simulink model "xpccanpcififo2"  (Simulink 4.00)
settings: Solver=FixedStepDiscrete  StartTime=0.0  StopTime=inf  RelTol=1e-3
libraries: xpclib x14, simulink3 x1
settings Model: Creator=mvetsch  LastModifiedBy=mvetsch  SimulationMode=external  RTWSystemTargetFile=xpctarget.tlc  RTWOptions="-aExtMode=1 -aForceParamTrailComments=0 -aInlineInvariantSignals=0 -aInlineParameters=0 -aLocalBlockOutputs=0 -aRL32IRQSourceModifier=\"Timer\" -aRL32LogBufSizeModifier=100000 -aRL32LogTETModifier=1 -aRL32ModeModifier=\"Real-Time\" -aRL32ObjectName=\"tg\" -aRL32ScopeModifier=1 -aRTWVerbose=1 -aRollThreshold=5 -aShowEliminatedStatements=1"  RTWTemplateMakefile=xpc_default_tmf  ExtModeMexFile=ext_xpc  ExtModeArmWhenConnect=off  OptimizeBlockIOStorage=off  BlockReductionOpt=off

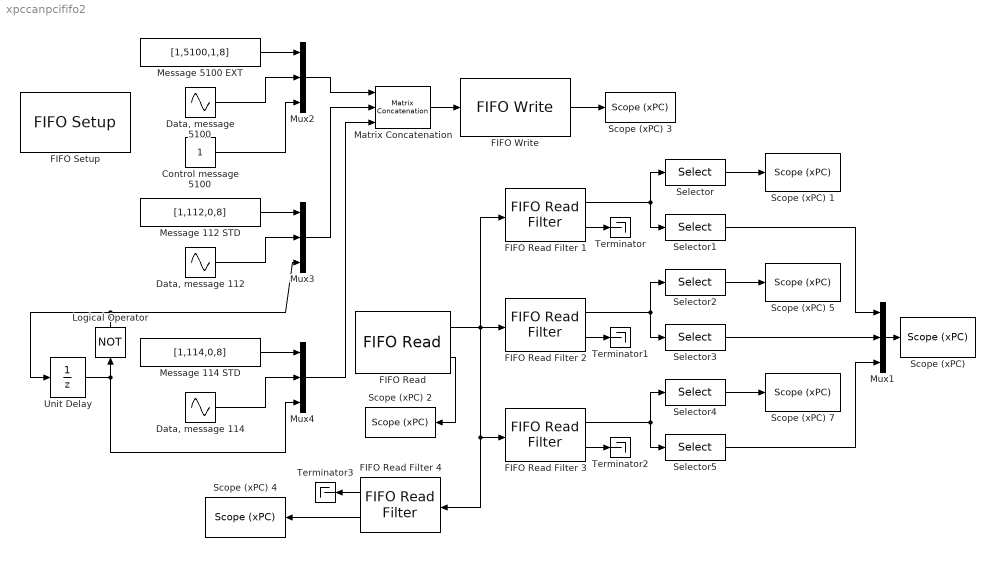
== system xpccanpcififo2 ==
  Control message 5100 : Constant  Value=1  VectorParams1D=off
  "Data, message 112" : Sin  Amplitude=2  Frequency=20*2*pi  Phase=0  SampleTime=0.001
  "Data, message 114" : Sin  Amplitude=3  Frequency=20*2*pi  Phase=0  SampleTime=0.001
  "Data, message 5100" : Sin  Amplitude=1  Frequency=20*2*pi  Phase=0  SampleTime=0.001
  "FIFO Read " : xpclib/CAN/Softing/CAN-AC2-PCI SJA 1000/FIFO Mode/FIFO Read   board=1  depth=3  status=on  sampletime=0.001
  FIFO Read Filter 1 : xpclib/CAN/Softing/CAN-AC2-PCI SJA 1000/FIFO Mode/FIFO Read Filter   portin=2  ctypein=EDF  direction=Include  ident=[5100]  identsel=Include
  FIFO Read Filter 2 : xpclib/CAN/Softing/CAN-AC2-PCI SJA 1000/FIFO Mode/FIFO Read Filter   portin=2  ctypein=SDF  direction=Include  ident=[112]  identsel=Include
  FIFO Read Filter 3 : xpclib/CAN/Softing/CAN-AC2-PCI SJA 1000/FIFO Mode/FIFO Read Filter   portin=2  ctypein=SDF  direction=Include  ident=[114]  identsel=Include
  FIFO Read Filter 4 : xpclib/CAN/Softing/CAN-AC2-PCI SJA 1000/FIFO Mode/FIFO Read Filter   Orientation=left  portin=2  ctypein=NE  direction=Include  ident=[]  identsel=Include
  "FIFO Setup " : xpclib/CAN/Softing/CAN-AC2-PCI SJA 1000/FIFO Mode/FIFO Setup   board=1  can1bus=Highspeed (ISO 11898)  can1Baudrate=1 MBaud  can1UserBR=[1,1,4,3]  acc1=[0,0,0,0]  can2bus=Highspeed (ISO 11898)  can2Baudrate=1 MBaud  can2UserBR=[1,1,4,3]  acc2=[0,0,0,0]  efdetection=off  init=[]  term=[]  ioBaseAddress=-1
  "FIFO Write " : xpclib/CAN/Softing/CAN-AC2-PCI SJA 1000/FIFO Mode/FIFO Write   board=1  status=on  sampletime=-1
  Logical Operator : Logic  Orientation=up  Operator=NOT  Inputs=2
  Matrix Concatenation : simulink3/Signals & Systems/Matrix Concatenation  numInports=3  catMethod=Vertical
  Message 112 STD : Constant  Value=[1,112,0,8]  VectorParams1D=off
  Message 114 STD : Constant  Value=[1,114,0,8]  VectorParams1D=off
  Message 5100 EXT : Constant  Value=[1,5100,1,8]  VectorParams1D=off
  Mux{1..4} (4 alike) : Mux  Inputs=3
  "Scope (xPC) " : xpclib/Misc./Scope (xPC)   scopeno=3  scopetype=Target  viewmode=Graphical redraw  grid=on  ylimits=[0,0]  autostart=on  nosamples=100  noprepostsamples=0  interleave=1  triggermode=FreeRun  triggersignal=1  triggerlevel=0.0  triggerslope=either  triggerscope=1
  Scope (xPC) 1 : xpclib/Misc./Scope (xPC)   scopeno=4  scopetype=Target  viewmode=Numerical  grid=on  ylimits=[0,0]  autostart=on  nosamples=3  noprepostsamples=0  interleave=1  triggermode=FreeRun  triggersignal=1  triggerlevel=0.0  triggerslope=either  triggerscope=1
  Scope (xPC) 2 : xpclib/Misc./Scope (xPC)   Orientation=left  scopeno=2  scopetype=Target  viewmode=Numerical  grid=on  ylimits=[0,0]  autostart=on  nosamples=3  noprepostsamples=0  interleave=1  triggermode=FreeRun  triggersignal=1  triggerlevel=0.0  triggerslope=either  triggerscope=1
  Scope (xPC) 3 : xpclib/Misc./Scope (xPC)   scopeno=1  scopetype=Target  viewmode=Numerical  grid=on  ylimits=[0,0]  autostart=on  nosamples=3  noprepostsamples=0  interleave=1  triggermode=FreeRun  triggersignal=1  triggerlevel=0.0  triggerslope=either  triggerscope=1
  Scope (xPC) 4 : xpclib/Misc./Scope (xPC)   Orientation=left  scopeno=7  scopetype=Target  viewmode=Numerical  grid=on  ylimits=[0,0]  autostart=on  nosamples=3  noprepostsamples=0  interleave=1  triggermode=FreeRun  triggersignal=1  triggerlevel=0.0  triggerslope=either  triggerscope=1
  Scope (xPC) 5 : xpclib/Misc./Scope (xPC)   scopeno=5  scopetype=Target  viewmode=Numerical  grid=on  ylimits=[0,0]  autostart=on  nosamples=3  noprepostsamples=0  interleave=1  triggermode=FreeRun  triggersignal=1  triggerlevel=0.0  triggerslope=either  triggerscope=1
  Scope (xPC) 7 : xpclib/Misc./Scope (xPC)   scopeno=6  scopetype=Target  viewmode=Numerical  grid=on  ylimits=[0,0]  autostart=on  nosamples=3  noprepostsamples=0  interleave=1  triggermode=FreeRun  triggersignal=1  triggerlevel=0.0  triggerslope=either  triggerscope=1
  Selector : Selector  InputType=Vector  ElementSrc=Internal  Elements=[1:5]  RowSrc=Internal  Rows=1  ColumnSrc=Internal  Columns=1  InputPortWidth=6
  Selector1 : Selector  InputType=Vector  ElementSrc=Internal  Elements=[6]  RowSrc=Internal  Rows=1  ColumnSrc=Internal  Columns=1  InputPortWidth=6
  Selector2 : Selector  InputType=Vector  ElementSrc=Internal  Elements=[1:5]  RowSrc=Internal  Rows=1  ColumnSrc=Internal  Columns=1  InputPortWidth=6
  Selector3 : Selector  InputType=Vector  ElementSrc=Internal  Elements=[6]  RowSrc=Internal  Rows=1  ColumnSrc=Internal  Columns=1  InputPortWidth=6
  Selector4 : Selector  InputType=Vector  ElementSrc=Internal  Elements=[1:5]  RowSrc=Internal  Rows=1  ColumnSrc=Internal  Columns=1  InputPortWidth=6
  Selector5 : Selector  InputType=Vector  ElementSrc=Internal  Elements=[6]  RowSrc=Internal  Rows=1  ColumnSrc=Internal  Columns=1  InputPortWidth=6
  Terminator{,1..3} (4 alike) : Terminator
  Unit Delay : UnitDelay  X0=0  SampleTime=0.001
  wires:
  Message 5100 EXT/1 -> Mux2/1
  "Data, message 5100"/1 -> Mux2/2
  "FIFO Read "/1 -> FIFO Read Filter 1/1, FIFO Read Filter 2/1, FIFO Read Filter 3/1, FIFO Read Filter 4/1
  "FIFO Read "/2 -> Scope (xPC) 2/1
  "FIFO Write "/1 -> Scope (xPC) 3/1
  Control message 5100/1 -> Mux2/3
  Unit Delay/1 -> Logical Operator/1, Mux4/3
  Logical Operator/1 -> Unit Delay/1, Mux3/3
  Message 112 STD/1 -> Mux3/1
  "Data, message 112"/1 -> Mux3/2
  Message 114 STD/1 -> Mux4/1
  "Data, message 114"/1 -> Mux4/2
  Mux3/1 -> Matrix Concatenation/2
  Mux2/1 -> Matrix Concatenation/1
  Mux4/1 -> Matrix Concatenation/3
  Matrix Concatenation/1 -> "FIFO Write "/1
  FIFO Read Filter 1/1 -> Selector/1, Selector1/1
  Selector/1 -> Scope (xPC) 1/1
  Selector2/1 -> Scope (xPC) 5/1
  Selector3/1 -> Mux1/2
  FIFO Read Filter 2/1 -> Selector2/1, Selector3/1
  Selector4/1 -> Scope (xPC) 7/1
  Selector5/1 -> Mux1/3
  FIFO Read Filter 3/1 -> Selector4/1, Selector5/1
  FIFO Read Filter 1/2 -> Terminator/1
  FIFO Read Filter 2/2 -> Terminator1/1
  FIFO Read Filter 3/2 -> Terminator2/1
  Selector1/1 -> Mux1/1
  Mux1/1 -> "Scope (xPC) "/1
  FIFO Read Filter 4/1 -> Terminator3/1
  FIFO Read Filter 4/2 -> Scope (xPC) 4/1
